simulink model "lookout"  (R2021a)
settings: Solver=VariableStepAuto  StartTime=0.0  StopTime=10.0  RelTol=1e-3
PreLoadFcn:
  | close all; clear all;
  | %% wczytanie danych
  | A = readmatrix('X[mm]_alfa[deg].txt');
  | X = A(:,1);
  | RAD = deg2rad(A(:,2));
libraries: simulink_extras x1
settings Model: Creator=micha  LastModifiedBy=micha

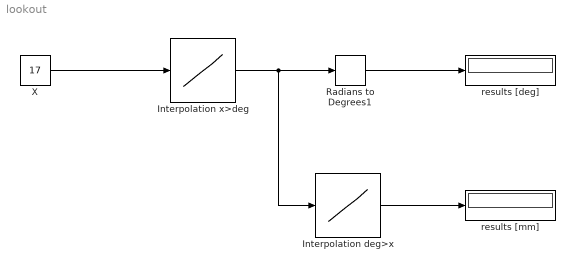
== system lookout ==
  Interpolation deg>x : Lookup_n-D  NumberOfTableDimensions=1  BreakpointsForDimension1=RAD  Table=X  InternalRulePriority=Speed  RndMeth=Simplest  InputSameDT=on
  Interpolation x>deg : Lookup_n-D  NumberOfTableDimensions=1  BreakpointsForDimension1=X  Table=RAD  InternalRulePriority=Speed  RndMeth=Simplest  InputSameDT=on
  Radians to Degrees1 : simulink_extras/Transformations/Radians to Degrees
  X : Constant  Value=17
  results [deg] : Display
  results [mm] : Display
  wires:
  X/1 -> Interpolation x>deg/1
  Interpolation x>deg/1 -> Radians to Degrees1/1, Interpolation deg>x/1
  Radians to Degrees1/1 -> results [deg]/1
  Interpolation deg>x/1 -> results [mm]/1
